simulink library "Energy_converter_Electrical_to_Mechanical"  (R2016a)
settings: Solver=ode1  StartTime=0.0  StopTime=Inf  FixedStep=0.001  RelTol=1e-3
undefined symbols (not defined in the file): API1dcac_efficiency, API2dcac_efficiency, API3dcac_efficiency, aux_power_state, AWR_InvStError, dat, DiscIntNeverNeededParam, EDCU_p_RefTqeMOT, emot_AcCmprFront_inertia, emot_AcCmprFront_nTab_3rdD, emot_AcCmprFront_pwrAC, emot_AcCmprFront_Tau, emot_AcCmprFront_trqTab_2ndD, emot_AcCmprFront_vltTab_1stD, emot_AcCmprRear_inertia, emot_AcCmprRear_nTab_3rdD, emot_AcCmprRear_pwrAC, emot_AcCmprRear_Tau, emot_AcCmprRear_trqTab_2ndD, emot_AcCmprRear_vltTab_1stD, emot_AirCmpr_inertia, emot_AirCmpr_nTab_3rdD, emot_AirCmpr_pwrAC, emot_AirCmpr_Tau, emot_AirCmpr_trqTab_2ndD, emot_AirCmpr_vltTab_1stD, emot_aircomp_power, emot_Cth_rotor, emot_Cth_stator, emot_dtrqEmotNeg, emot_dtrqEmotPtv, emot_inv_pwracTab_1st, emot_inv_pwrDC, emot_inv_pwrLoss, emot_inv_VrmsTab_2nd, emot_j, emot_mot_pwrLoss, emot_nTab_1stD, emot_pwrEtaTab_nRow, emot_pwrEtaTab_pwrTab, emot_pwrEtaTab_trqClm, emot_Rth_rotor_oil, emot_Rth_stator_oil, emot_Rth_stator_rotor, emot_tractiongroup, emot_Trotor_init, emot_trqMaxRow, emot_trqMinRow, emot_Tstator_init, emot_vltTab_3rdD, FirstDrivenAxleNoOfEmot, inv_Cth_cooling_plate, inv_Cth_diode, inv_Cth_IGBT, inv_n_IGBT_per_Switch, inv_Rth_cooling_plate_coolant, inv_Rth_PS_cooling_plate, inv_Tplate_init, inv_Tpowerstack_init, midAxleNoOfEmot ... (+6)
libraries: Electrical_converter x12, Energy_converter_Electrical_to_Mechanical x12, simulink x7
(part 5 of 8)

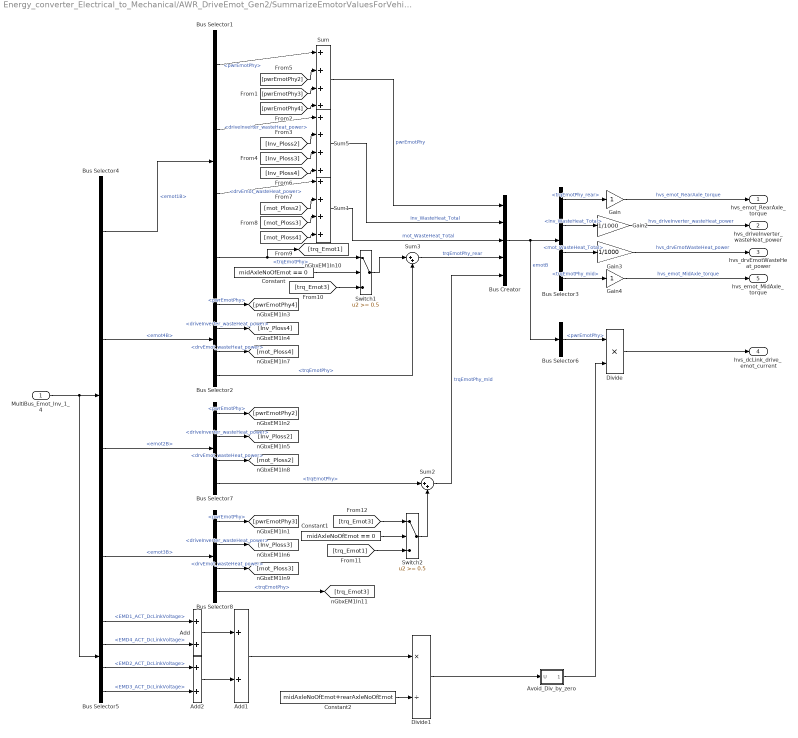
== system Energy_converter_Electrical_to_Mechanical/AWR_DriveEmot_Gen2/SummarizeEmotorValuesForVehicle ==
  MultiBus_Emot_Inv_1_4 : Inport
  Add : Sum
  Add1 : Sum
  Add2 : Sum
  Avoid_Div_by_zero : Subsystem
  Bus Creator : BusCreator  Inputs=5
  Bus Selector{1..2,7..8} (4 alike) : BusSelector  OutputSignals=pwrEmotPhy,driveInverter_wasteHeat_power,drvEmot_wasteHeat_power,trqEmotPhy
  Bus Selector3 : BusSelector  OutputSignals=trqEmotPhy_rear,Inv_WasteHeat_Total,mot_WasteHeat_Total,trqEmotPhy_mid
  Bus Selector4 : BusSelector  OutputSignals=emot1_4B.emot1B,emot1_4B.emot4B,emot2_3B.emot2B,emot2_3B.emot3B
  Bus Selector5 : BusSelector  OutputSignals=awr1_4B.awr1B.EMD1_ACT_DcLinkVoltage,awr1_4B.awr4B.EMD4_ACT_DcLinkVoltage,awr2_3B.awr2B.EMD2_ACT_DcLinkVoltage,awr2_3B.awr3B.EMD3_ACT_DcLinkVoltage
  Bus Selector6 : BusSelector  OutputSignals=pwrEmotPhy
  Constant : Constant  Value=midAxleNoOfEmot == 0
  Constant1 : Constant  Value=midAxleNoOfEmot == 0
  Constant2 : Constant  Value=midAxleNoOfEmot+rearAxleNoOfEmot
  Divide : Product  Inputs=**
  Divide1 : Product  Inputs=*/
  Gain : Gain
  Gain2 : Gain  Gain=1/1000
  Gain3 : Gain  Gain=1/1000
  Gain4 : Gain
  Sum : Sum  Inputs=|++++
  Sum1 : Sum  Inputs=|++++
  Sum2 : Sum  Inputs=|++
  Sum3 : Sum  Inputs=|++
  Sum5 : Sum  Inputs=|++++
  Switch1 : Switch  Threshold=0.5
  Switch2 : Switch  Threshold=0.5
  hvs_emot_RearAxle_torque : Outport
  hvs_driveInverter_wasteHeat_power : Outport  Port=2
  hvs_drvEmotWasteHeat_power : Outport  Port=3
  hvs_dcLink_drive_emot_current : Outport  Port=4
  hvs_emot_MidAxle_torque : Outport  Port=5
  wires:
  Add1/1 -> Divide1/1
  Constant2/1 -> Divide1/2
  [trq_Emot3] -> Switch2/1
  Switch2/1 -> Sum2/2
  [trq_Emot1] -> Switch2/3
  Constant1/1 -> Switch2/2
  [trq_Emot3] -> Switch1/3
  Switch1/1 -> Sum3/1
  Constant/1 -> Switch1/2
  Sum3/1 -> Bus Creator/4  "trqEmotPhy_rear"
  Sum1/1 -> Bus Creator/3  "mot_WasteHeat_Total"
  Sum5/1 -> Bus Creator/2  "Inv_WasteHeat_Total"
  Sum/1 -> Bus Creator/1  "pwrEmotPhy"
  Bus Selector2/4 -> Sum3/2  "<trqEmotPhy>"
  Bus Selector1/4 -> Switch1/1, [trq_Emot1]  "<trqEmotPhy>"
  Bus Selector2/3 -> [mot_Ploss4]  "<drvEmot_wasteHeat_power>"
  Bus Selector2/2 -> [Inv_Ploss4]  "<driveInverter_wasteHeat_power>"
  Bus Selector1/1 -> Sum/1  "<pwrEmotPhy>"
  Bus Selector4/2 -> Bus Selector2/1  "<emot4B>"
  Bus Selector4/1 -> Bus Selector1/1  "<emot1B>"
  MultiBus_Emot_Inv_1_4/1 -> Bus Selector5/1, Bus Selector4/1
  Bus Creator/1 -> Bus Selector6/1, Bus Selector3/1  "emotB"
  Bus Selector3/1 -> Gain/1  "<trqEmotPhy_rear>"
  Gain/1 -> hvs_emot_RearAxle_torque/1  "hvs_emot_RearAxle_torque"
  Bus Selector5/1 -> Add/1  "<EMD1_ACT_DcLinkVoltage>"
  Bus Selector5/2 -> Add/2  "<EMD4_ACT_DcLinkVoltage>"
  Divide1/1 -> Avoid_Div_by_zero/1(U)
  Bus Selector6/1 -> Divide/1  "<pwrEmotPhy>"
  Avoid_Div_by_zero/1(1/U) -> Divide/2
  Divide/1 -> hvs_dcLink_drive_emot_current/1
  Bus Selector3/2 -> Gain2/1  "<Inv_WasteHeat_Total>"
  Gain2/1 -> hvs_driveInverter_wasteHeat_power/1  "hvs_driveInverter_wasteHeat_power"
  Bus Selector3/3 -> Gain3/1  "<mot_WasteHeat_Total>"
  Gain3/1 -> hvs_drvEmotWasteHeat_power/1  "hvs_drvEmotWasteHeat_power"
  Bus Selector4/4 -> Bus Selector8/1  "<emot3B>"
  Bus Selector4/3 -> Bus Selector7/1  "<emot2B>"
  Bus Selector7/1 -> [pwrEmotPhy2]  "<pwrEmotPhy>"
  Bus Selector8/1 -> [pwrEmotPhy3]  "<pwrEmotPhy>"
  Bus Selector2/1 -> [pwrEmotPhy4]  "<pwrEmotPhy>"
  [pwrEmotPhy2] -> Sum/2
  [pwrEmotPhy3] -> Sum/3
  [pwrEmotPhy4] -> Sum/4
  [Inv_Ploss2] -> Sum5/2
  [Inv_Ploss3] -> Sum5/3
  [Inv_Ploss4] -> Sum5/4
  Bus Selector7/2 -> [Inv_Ploss2]  "<driveInverter_wasteHeat_power>"
  Bus Selector8/2 -> [Inv_Ploss3]  "<driveInverter_wasteHeat_power>"
  Bus Selector7/3 -> [mot_Ploss2]  "<drvEmot_wasteHeat_power>"
  Bus Selector8/3 -> [mot_Ploss3]  "<drvEmot_wasteHeat_power>"
  [mot_Ploss2] -> Sum1/2
  [mot_Ploss3] -> Sum1/3
  [mot_Ploss4] -> Sum1/4
  Bus Selector7/4 -> Sum2/1  "<trqEmotPhy>"
  Bus Selector8/4 -> [trq_Emot3]  "<trqEmotPhy>"
  Sum2/1 -> Bus Creator/5  "trqEmotPhy_mid"
  Bus Selector5/3 -> Add2/1  "<EMD2_ACT_DcLinkVoltage>"
  Bus Selector5/4 -> Add2/2  "<EMD3_ACT_DcLinkVoltage>"
  Gain4/1 -> hvs_emot_MidAxle_torque/1  "hvs_emot_MidAxle_torque"
  Bus Selector3/4 -> Gain4/1  "<trqEmotPhy_mid>"
  Add/1 -> Add1/1
  Add2/1 -> Add1/2
  Bus Selector1/2 -> Sum5/1  "<driveInverter_wasteHeat_power>"
  Bus Selector1/3 -> Sum1/1  "<drvEmot_wasteHeat_power>"

== system Energy_converter_Electrical_to_Mechanical/AWR_DriveEmot_Gen2/percent_to_Nm ==
  Percentage_Torque : Inport
  Reference_Torque : Inport  Port=2
  Constant : Constant  Value=100
  Divide : Product  Inputs=*/
  Product : Product  RndMeth=Zero
  Torque_Nm : Outport
  wires:
  Constant/1 -> Divide/2
  Product/1 -> Divide/1
  Reference_Torque/1 -> Product/2  "Reference_Torque"
  Divide/1 -> Torque_Nm/1  "Torque_Nm"
  Percentage_Torque/1 -> Product/1  "Percentage_Torque"

== system Energy_converter_Electrical_to_Mechanical/AWR_DriveEmot_Gen2/percent_to_Nm1 ==
  Percentage_Torque : Inport
  Reference_Torque : Inport  Port=2
  Constant : Constant  Value=100
  Divide : Product  Inputs=*/
  Product : Product  RndMeth=Zero
  Torque_Nm : Outport
  wires:
  Constant/1 -> Divide/2
  Product/1 -> Divide/1
  Reference_Torque/1 -> Product/2  "Reference_Torque"
  Divide/1 -> Torque_Nm/1  "Torque_Nm"
  Percentage_Torque/1 -> Product/1  "Percentage_Torque"

== system Energy_converter_Electrical_to_Mechanical/AWR_DriveEmot_Gen2/percent_to_Nm2 ==
  Percentage_Torque : Inport
  Reference_Torque : Inport  Port=2
  Constant : Constant  Value=100
  Divide : Product  Inputs=*/
  Product : Product  RndMeth=Zero
  Torque_Nm : Outport
  wires:
  Constant/1 -> Divide/2
  Product/1 -> Divide/1
  Reference_Torque/1 -> Product/2  "Reference_Torque"
  Divide/1 -> Torque_Nm/1  "Torque_Nm"
  Percentage_Torque/1 -> Product/1  "Percentage_Torque"

== system Energy_converter_Electrical_to_Mechanical/AWR_DriveEmot_Gen2/percent_to_Nm3 ==
  Percentage_Torque : Inport
  Reference_Torque : Inport  Port=2
  Constant : Constant  Value=100
  Divide : Product  Inputs=*/
  Product : Product  RndMeth=Zero
  Torque_Nm : Outport
  wires:
  Constant/1 -> Divide/2
  Product/1 -> Divide/1
  Reference_Torque/1 -> Product/2  "Reference_Torque"
  Divide/1 -> Torque_Nm/1  "Torque_Nm"
  Percentage_Torque/1 -> Product/1  "Percentage_Torque"

== system Energy_converter_Electrical_to_Mechanical/AWR_DriveEmot_edb_Data/AWR 1 TX ==
  IN_EMD1_ACT_DcLinkVoltage : Inport
  IN_EMD1_ACT_DigitalInput1 : Inport  Port=2
  IN_EMD1_ACT_MaximumAvailableTorque : Inport  Port=3
  IN_EMD1_ACT_DcLinkPower : Inport  Port=4
  IN_EMD1_ACT_MotorSpeed : Inport  Port=5
  IN_EMD1_ACT_Torque : Inport  Port=6
  IN_EMD1_ACT_InverterState : Inport  Port=7
  IN_EMD1_ACT_ReferenceTorqueLimited : Inport  Port=8
  IN_EMD1_ACT_MaxJunctionTemperature : Inport  Port=9
  IN_EMD1_ACT_MotorTemperature : Inport  Port=10
  IN_EMD1_ACT_InverterLosses : Inport  Port=11
  IN_EMD1_ACT_MotorLosses : Inport  Port=12
  Constant3 : Constant  Value=EDCU_p_RefTqeMOT
  Constant39 : Constant  Value=EDCU_p_RefTqeMOT
  Constant5 : Constant  Value=EDCU_p_RefTqeMOT
  Nm_to_percent : Subsystem
  Nm_to_percent1 : Subsystem
  Nm_to_percent2 : Subsystem
  hvs_EMD1_ACT_DigitalInput1 : Outport
  hvs_EMD1_ACT_InverterState : Outport  Port=2
  hvs_EMD1_ACT_MaxAvailableTorque : Outport  Port=3
  hvs_EMD1_ACT_ReferenceTorqueLim : Outport  Port=4
  hvs_EMD1_ACT_Torque : Outport  Port=5
  hvs_EMD1_ACT_DcLinkPower : Outport  Port=6
  hvs_EMD1_ACT_MotorSpeed : Outport  Port=7
  hvs_EMD1_ACT_DcLinkVoltage : Outport  Port=8
  hvs_EMD1_ACT_MaxJunctionTemp : Outport  Port=9
  hvs_EMD1_ACT_MotorTemperature : Outport  Port=10
  hvs_EMD1_ACT_InverterLosses : Outport  Port=11
  hvs_EMD1_ACT_MotorLosses : Outport  Port=12
  wires:
  Constant5/1 -> Nm_to_percent1/2(Reference_Torque)
  IN_EMD1_ACT_ReferenceTorqueLimited/1 -> Nm_to_percent1/1(Nm_Torque)  "EMD1_ACT_ReferenceTorqueLimited"
  IN_EMD1_ACT_InverterState/1 -> hvs_EMD1_ACT_InverterState/1  "hvs_EMD1_ACT_InverterState"
  IN_EMD1_ACT_DcLinkPower/1 -> hvs_EMD1_ACT_DcLinkPower/1  "hvs_EMD1_ACT_DcLinkPower"
  IN_EMD1_ACT_DcLinkVoltage/1 -> hvs_EMD1_ACT_DcLinkVoltage/1  "hvs_EMD1_ACT_DcLinkVoltage"
  Nm_to_percent/1(Torque_Percentage) -> hvs_EMD1_ACT_MaxAvailableTorque/1  "hvs_EMD1_ACT_MaxAvailableTorque"
  Nm_to_percent1/1(Torque_Percentage) -> hvs_EMD1_ACT_ReferenceTorqueLim/1  "hvs_EMD1_ACT_ReferenceTorqueLim"
  IN_EMD1_ACT_MotorSpeed/1 -> hvs_EMD1_ACT_MotorSpeed/1  "hvs_EMD1_ACT_MotorSpeed"
  IN_EMD1_ACT_Torque/1 -> Nm_to_percent2/1(Nm_Torque)
  IN_EMD1_ACT_MaxJunctionTemperature/1 -> hvs_EMD1_ACT_MaxJunctionTemp/1  "hvs_EMD1_ACT_MaxJunctionTemp"
  IN_EMD1_ACT_MotorTemperature/1 -> hvs_EMD1_ACT_MotorTemperature/1  "hvs_EMD1_ACT_MotorTemperature"
  IN_EMD1_ACT_DigitalInput1/1 -> hvs_EMD1_ACT_DigitalInput1/1  "hvs_EMD1_ACT_DigitalInput1"
  IN_EMD1_ACT_MaximumAvailableTorque/1 -> Nm_to_percent/1(Nm_Torque)  "EMD1_ACT_MaximumAvailableTorque"
  Constant3/1 -> Nm_to_percent/2(Reference_Torque)
  Nm_to_percent2/1(Torque_Percentage) -> hvs_EMD1_ACT_Torque/1  "hvs_EMD1_ACT_Torque"
  Constant39/1 -> Nm_to_percent2/2(Reference_Torque)
  IN_EMD1_ACT_InverterLosses/1 -> hvs_EMD1_ACT_InverterLosses/1  "hvs_EMD1_ACT_InverterLosses"
  IN_EMD1_ACT_MotorLosses/1 -> hvs_EMD1_ACT_MotorLosses/1  "hvs_EMD1_ACT_MotorLosses"

== system Energy_converter_Electrical_to_Mechanical/AWR_DriveEmot_edb_Data/AWR 2 TX ==
  IN_EMD2_ACT_DcLinkVoltage : Inport
  IN_EMD2_ACT_DigitalInput1 : Inport  Port=2
  IN_EMD2_ACT_MaximumAvailableTorque : Inport  Port=3
  IN_EMD2_ACT_DcLinkPower : Inport  Port=4
  IN_EMD2_ACT_MotorSpeed : Inport  Port=5
  IN_EMD2_ACT_Torque : Inport  Port=6
  IN_EMD2_ACT_InverterState : Inport  Port=7
  IN_EMD2_ACT_ReferenceTorqueLimited : Inport  Port=8
  IN_EMD2_ACT_MaxJunctionTemperature : Inport  Port=9
  IN_EMD2_ACT_MotorTemperature : Inport  Port=10
  IN_EMD2_ACT_InverterLosses : Inport  Port=11
  IN_EMD2_ACT_MotorLosses : Inport  Port=12
  Constant3 : Constant  Value=EDCU_p_RefTqeMOT
  Constant39 : Constant  Value=EDCU_p_RefTqeMOT
  Constant5 : Constant  Value=EDCU_p_RefTqeMOT
  Nm_to_percent : Subsystem
  Nm_to_percent1 : Subsystem
  Nm_to_percent2 : Subsystem
  hvs_EMD2_ACT_DigitalInput1 : Outport
  hvs_EMD2_ACT_InverterState : Outport  Port=2
  hvs_EMD2_ACT_MaxAvailableTorque : Outport  Port=3
  hvs_EMD2_ACT_ReferenceTorqueLim : Outport  Port=4
  hvs_EMD2_ACT_Torque : Outport  Port=5
  hvs_EMD2_ACT_DcLinkPower : Outport  Port=6
  hvs_EMD2_ACT_MotorSpeed : Outport  Port=7
  hvs_EMD2_ACT_DcLinkVoltage : Outport  Port=8
  hvs_EMD2_ACT_MaxJunctionTemp : Outport  Port=9
  hvs_EMD2_ACT_MotorTemperature : Outport  Port=10
  hvs_EMD2_ACT_InverterLosses : Outport  Port=11
  hvs_EMD2_ACT_MotorLosses : Outport  Port=12
  wires:
  Constant5/1 -> Nm_to_percent1/2(Reference_Torque)
  IN_EMD2_ACT_ReferenceTorqueLimited/1 -> Nm_to_percent1/1(Nm_Torque)  "EMD1_ACT_ReferenceTorqueLimited"
  IN_EMD2_ACT_InverterState/1 -> hvs_EMD2_ACT_InverterState/1  "hvs_EMD2_ACT_InverterState"
  IN_EMD2_ACT_DcLinkPower/1 -> hvs_EMD2_ACT_DcLinkPower/1  "hvs_EMD2_ACT_DcLinkPower"
  IN_EMD2_ACT_DcLinkVoltage/1 -> hvs_EMD2_ACT_DcLinkVoltage/1  "hvs_EMD2_ACT_DcLinkVoltage"
  Nm_to_percent/1(Torque_Percentage) -> hvs_EMD2_ACT_MaxAvailableTorque/1  "hvs_EMD2_ACT_MaxAvailableTorque"
  Nm_to_percent1/1(Torque_Percentage) -> hvs_EMD2_ACT_ReferenceTorqueLim/1  "hvs_EMD2_ACT_ReferenceTorqueLim"
  IN_EMD2_ACT_MotorSpeed/1 -> hvs_EMD2_ACT_MotorSpeed/1  "hvs_EMD2_ACT_MotorSpeed"
  IN_EMD2_ACT_Torque/1 -> Nm_to_percent2/1(Nm_Torque)
  IN_EMD2_ACT_MaxJunctionTemperature/1 -> hvs_EMD2_ACT_MaxJunctionTemp/1  "hvs_EMD2_ACT_MaxJunctionTemp"
  IN_EMD2_ACT_MotorTemperature/1 -> hvs_EMD2_ACT_MotorTemperature/1  "hvs_EMD2_ACT_MotorTemperature"
  IN_EMD2_ACT_DigitalInput1/1 -> hvs_EMD2_ACT_DigitalInput1/1  "hvs_EMD2_ACT_DigitalInput1"
  IN_EMD2_ACT_MaximumAvailableTorque/1 -> Nm_to_percent/1(Nm_Torque)  "EMD1_ACT_MaximumAvailableTorque"
  Constant3/1 -> Nm_to_percent/2(Reference_Torque)
  Nm_to_percent2/1(Torque_Percentage) -> hvs_EMD2_ACT_Torque/1  "hvs_EMD2_ACT_Torque"
  Constant39/1 -> Nm_to_percent2/2(Reference_Torque)
  IN_EMD2_ACT_InverterLosses/1 -> hvs_EMD2_ACT_InverterLosses/1  "hvs_EMD2_ACT_InverterLosses"
  IN_EMD2_ACT_MotorLosses/1 -> hvs_EMD2_ACT_MotorLosses/1  "hvs_EMD2_ACT_MotorLosses"

== system Energy_converter_Electrical_to_Mechanical/AWR_DriveEmot_edb_Data/AWR 3 TX ==
  IN_EMD3_ACT_DcLinkVoltage : Inport
  IN_EMD3_ACT_DigitalInput1 : Inport  Port=2
  IN_EMD3_ACT_MaximumAvailableTorque : Inport  Port=3
  IN_EMD3_ACT_DcLinkPower : Inport  Port=4
  IN_EMD3_ACT_MotorSpeed : Inport  Port=5
  IN_EMD3_ACT_Torque : Inport  Port=6
  IN_EMD3_ACT_InverterState : Inport  Port=7
  IN_EMD3_ACT_ReferenceTorqueLimited : Inport  Port=8
  IN_EMD3_ACT_MaxJunctionTemperature : Inport  Port=9
  IN_EMD3_ACT_MotorTemperature : Inport  Port=10
  IN_EMD3_ACT_InverterLosses : Inport  Port=11
  IN_EMD3_ACT_MotorLosses : Inport  Port=12
  Constant3 : Constant  Value=EDCU_p_RefTqeMOT
  Constant39 : Constant  Value=EDCU_p_RefTqeMOT
  Constant5 : Constant  Value=EDCU_p_RefTqeMOT
  Nm_to_percent : Subsystem
  Nm_to_percent1 : Subsystem
  Nm_to_percent2 : Subsystem
  hvs_EMD3_ACT_DigitalInput1 : Outport
  hvs_EMD3_ACT_InverterState : Outport  Port=2
  hvs_EMD3_ACT_MaxAvailableTorque : Outport  Port=3
  hvs_EMD3_ACT_ReferenceTorqueLim : Outport  Port=4
  hvs_EMD3_ACT_Torque : Outport  Port=5
  hvs_EMD3_ACT_DcLinkPower : Outport  Port=6
  hvs_EMD3_ACT_MotorSpeed : Outport  Port=7
  hvs_EMD3_ACT_DcLinkVoltage : Outport  Port=8
  hvs_EMD3_ACT_MaxJunctionTemp : Outport  Port=9
  hvs_EMD3_ACT_MotorTemperature : Outport  Port=10
  hvs_EMD3_ACT_InverterLosses : Outport  Port=11
  hvs_EMD3_ACT_MotorLosses : Outport  Port=12
  wires:
  Constant39/1 -> Nm_to_percent2/2(Reference_Torque)
  Nm_to_percent2/1(Torque_Percentage) -> hvs_EMD3_ACT_Torque/1  "hvs_EMD3_ACT_Torque"
  Constant3/1 -> Nm_to_percent/2(Reference_Torque)
  IN_EMD3_ACT_MaximumAvailableTorque/1 -> Nm_to_percent/1(Nm_Torque)  "EMD1_ACT_MaximumAvailableTorque"
  IN_EMD3_ACT_DigitalInput1/1 -> hvs_EMD3_ACT_DigitalInput1/1  "hvs_EMD3_ACT_DigitalInput1"
  IN_EMD3_ACT_MotorTemperature/1 -> hvs_EMD3_ACT_MotorTemperature/1  "hvs_EMD3_ACT_MotorTemperature"
  IN_EMD3_ACT_MaxJunctionTemperature/1 -> hvs_EMD3_ACT_MaxJunctionTemp/1  "hvs_EMD3_ACT_MaxJunctionTemp"
  IN_EMD3_ACT_Torque/1 -> Nm_to_percent2/1(Nm_Torque)
  IN_EMD3_ACT_MotorSpeed/1 -> hvs_EMD3_ACT_MotorSpeed/1  "hvs_EMD3_ACT_MotorSpeed"
  Nm_to_percent1/1(Torque_Percentage) -> hvs_EMD3_ACT_ReferenceTorqueLim/1  "hvs_EMD3_ACT_ReferenceTorqueLim"
  Nm_to_percent/1(Torque_Percentage) -> hvs_EMD3_ACT_MaxAvailableTorque/1  "hvs_EMD3_ACT_MaxAvailableTorque"
  IN_EMD3_ACT_DcLinkVoltage/1 -> hvs_EMD3_ACT_DcLinkVoltage/1  "hvs_EMD3_ACT_DcLinkVoltage"
  IN_EMD3_ACT_DcLinkPower/1 -> hvs_EMD3_ACT_DcLinkPower/1  "hvs_EMD3_ACT_DcLinkPower"
  IN_EMD3_ACT_InverterState/1 -> hvs_EMD3_ACT_InverterState/1  "hvs_EMD3_ACT_InverterState"
  IN_EMD3_ACT_ReferenceTorqueLimited/1 -> Nm_to_percent1/1(Nm_Torque)  "EMD1_ACT_ReferenceTorqueLimited"
  Constant5/1 -> Nm_to_percent1/2(Reference_Torque)
  IN_EMD3_ACT_InverterLosses/1 -> hvs_EMD3_ACT_InverterLosses/1  "hvs_EMD3_ACT_InverterLosses"
  IN_EMD3_ACT_MotorLosses/1 -> hvs_EMD3_ACT_MotorLosses/1  "hvs_EMD3_ACT_MotorLosses"

== system Energy_converter_Electrical_to_Mechanical/AWR_DriveEmot_edb_Data/AWR 4 TX ==
  IN_EMD4_ACT_DcLinkVoltage : Inport
  IN_EMD4_ACT_DigitalInput1 : Inport  Port=2
  IN_EMD4_ACT_MaximumAvailableTorque : Inport  Port=3
  IN_EMD4_ACT_DcLinkPower : Inport  Port=4
  IN_EMD4_ACT_MotorSpeed : Inport  Port=5
  IN_EMD4_ACT_Torque : Inport  Port=6
  IN_EMD4_ACT_InverterState : Inport  Port=7
  IN_EMD4_ACT_ReferenceTorqueLimited : Inport  Port=8
  IN_EMD4_ACT_MaxJunctionTemperature : Inport  Port=9
  IN_EMD4_ACT_MotorTemperature : Inport  Port=10
  IN_EMD4_ACT_InverterLosses : Inport  Port=11
  IN_EMD4_ACT_MotorLosses : Inport  Port=12
  Constant3 : Constant  Value=EDCU_p_RefTqeMOT
  Constant39 : Constant  Value=EDCU_p_RefTqeMOT
  Constant5 : Constant  Value=EDCU_p_RefTqeMOT
  Nm_to_percent : Subsystem
  Nm_to_percent1 : Subsystem
  Nm_to_percent2 : Subsystem
  hvs_EMD4_ACT_DigitalInput1 : Outport
  hvs_EMD4_ACT_InverterState : Outport  Port=2
  hvs_EMD4_ACT_MaxAvailableTorque : Outport  Port=3
  hvs_EMD4_ACT_ReferenceTorqueLim : Outport  Port=4
  hvs_EMD4_ACT_Torque : Outport  Port=5
  hvs_EMD4_ACT_DcLinkPower : Outport  Port=6
  hvs_EMD4_ACT_MotorSpeed : Outport  Port=7
  hvs_EMD4_ACT_DcLinkVoltage : Outport  Port=8
  hvs_EMD4_ACT_MaxJunctionTemperature : Outport  Port=9
  hvs_EMD4_ACT_MotorTemperature : Outport  Port=10
  hvs_EMD4_ACT_InverterLosses : Outport  Port=11
  hvs_EMD4_ACT_MotorLosses : Outport  Port=12
  wires:
  Constant5/1 -> Nm_to_percent1/2(Reference_Torque)
  IN_EMD4_ACT_ReferenceTorqueLimited/1 -> Nm_to_percent1/1(Nm_Torque)  "EMD4_ACT_ReferenceTorqueLimited"
  IN_EMD4_ACT_InverterState/1 -> hvs_EMD4_ACT_InverterState/1  "hvs_EMD4_ACT_InverterState"
  IN_EMD4_ACT_DcLinkPower/1 -> hvs_EMD4_ACT_DcLinkPower/1  "hvs_EMD4_ACT_DcLinkPower"
  IN_EMD4_ACT_DcLinkVoltage/1 -> hvs_EMD4_ACT_DcLinkVoltage/1  "hvs_EMD4_ACT_DcLinkVoltage"
  Nm_to_percent/1(Torque_Percentage) -> hvs_EMD4_ACT_MaxAvailableTorque/1  "hvs_EMD4_ACT_MaxAvailableTorque"
  IN_EMD4_ACT_MotorSpeed/1 -> hvs_EMD4_ACT_MotorSpeed/1  "hvs_EMD4_ACT_MotorSpeed"
  IN_EMD4_ACT_Torque/1 -> Nm_to_percent2/1(Nm_Torque)
  IN_EMD4_ACT_MaxJunctionTemperature/1 -> hvs_EMD4_ACT_MaxJunctionTemperature/1  "hvs_EMD4_ACT_MaxJunctionTemperature"
  IN_EMD4_ACT_MotorTemperature/1 -> hvs_EMD4_ACT_MotorTemperature/1  "hvs_EMD4_ACT_MotorTemperature"
  Nm_to_percent1/1(Torque_Percentage) -> hvs_EMD4_ACT_ReferenceTorqueLim/1  "hvs_EMD4_ACT_ReferenceTorqueLim"
  IN_EMD4_ACT_DigitalInput1/1 -> hvs_EMD4_ACT_DigitalInput1/1  "hvs_EMD4_ACT_DigitalInput1"
  IN_EMD4_ACT_MaximumAvailableTorque/1 -> Nm_to_percent/1(Nm_Torque)  "EMD2_ACT_MaximumAvailableTorque"
  Constant3/1 -> Nm_to_percent/2(Reference_Torque)
  Constant39/1 -> Nm_to_percent2/2(Reference_Torque)
  Nm_to_percent2/1(Torque_Percentage) -> hvs_EMD4_ACT_Torque/1  "hvs_EMD4_ACT_Torque"
  IN_EMD4_ACT_InverterLosses/1 -> hvs_EMD4_ACT_InverterLosses/1  "hvs_EMD4_ACT_InverterLosses"
  IN_EMD4_ACT_MotorLosses/1 -> hvs_EMD4_ACT_MotorLosses/1  "hvs_EMD4_ACT_MotorLosses"

== system Energy_converter_Electrical_to_Mechanical/AWR_DriveEmot_edb_Data/AWR1_4 ==
  EMD1_CMD_Commamd : Inport
  EMD1_CMD_MotorControlMode : Inport  Port=2
  EMD1_CMD_SpeedRefLim : Inport  Port=3
  EMD1_CMD_TorqueRefLim : Inport  Port=4
  HVFreigabeHW_SiRelay_D : Inport  Port=5
  vltZkBmsPhy : Inport  Port=6
  trqEmot1Phy : Inport  Port=7
  trqEmot4Phy : Inport  Port=8
  pwEmot1Phy : Inport  Port=9
  pwEmot4Phy : Inport  Port=10
  trqEmot1Max : Inport  Port=11
  trqEmot4Max : Inport  Port=12
  nGbxEMIn : Inport  Port=13
  EMD4_CMD_Commamd : Inport  Port=14
  EMD4_CMD_MotorControlMode : Inport  Port=15
  EMD4_CMD_SpeedRefLim : Inport  Port=16
  EMD4_CMD_TorqueRefLim : Inport  Port=17
  HVFreigabeHW4_SiRelay_D : Inport  Port=18
  EDCU_Dig_SafetyCutOffDG1 : Inport  Port=19
  Bus Creator3 : BusCreator  Inputs=11
  Bus Creator4 : BusCreator  Inputs=2
  Bus Creator5 : BusCreator  Inputs=11
  Gain : Gain
  Gain1 : Gain
  Switch1 : Switch  Threshold=0.5
  Switch2 : Switch  Threshold=0.5
  ZeroWhenNotReady1 : Subsystem  TreatAsAtomicUnit=on
  ZeroWhenNotReady2 : Subsystem  TreatAsAtomicUnit=on
  awr : Electrical_converter/awr  SystemSampleTime=-1
  awr1 : Electrical_converter/awr  SystemSampleTime=-1
  awr1_4B : Outport
  wires:
  nGbxEMIn/1 -> [nGbxEMIn], awr/10
  vltZkBmsPhy/1 -> [vltZkBmsPhy], awr/6
  EMD1_CMD_MotorControlMode/1 -> awr/2
  EMD4_CMD_MotorControlMode/1 -> awr1/2
  [nGbxEMIn] -> awr1/10
  Gain1/1 -> Bus Creator3/1  "EMD4_ACT_DcLinkVoltage"
  Gain/1 -> Bus Creator5/1  "EMD1_ACT_DcLinkVoltage"
  EMD1_CMD_SpeedRefLim/1 -> awr/3
  EMD1_CMD_TorqueRefLim/1 -> awr/4
  HVFreigabeHW_SiRelay_D/1 -> awr/5
  HVFreigabeHW4_SiRelay_D/1 -> awr1/5
  EMD4_CMD_SpeedRefLim/1 -> awr1/3
  EMD4_CMD_Commamd/1 -> awr1/1
  EMD4_CMD_TorqueRefLim/1 -> awr1/4
  Bus Creator4/1 -> awr1_4B/1  "awr1_4B"
  trqEmot4Phy/1 -> awr1/7
  pwEmot4Phy/1 -> awr1/8
  trqEmot4Max/1 -> awr1/9
  trqEmot1Phy/1 -> awr/7
  pwEmot1Phy/1 -> awr/8
  trqEmot1Max/1 -> awr/9
  Bus Creator3/1 -> Switch1/1  "awr4B"
  ZeroWhenNotReady2/1(Out1) -> Switch1/3
  Switch1/1 -> Bus Creator4/2  "awr4B"
  awr1/2 -> Bus Creator3/2
  awr1/3 -> Bus Creator3/3
  awr1/10 -> Bus Creator3/10
  awr1/11 -> Bus Creator3/11
  awr1/5 -> Bus Creator3/5
  awr1/9 -> Bus Creator3/9
  awr1/8 -> Bus Creator3/8
  awr1/7 -> Bus Creator3/7
  awr1/6 -> Bus Creator3/6
  awr1/1 -> Gain1/1
  awr1/4 -> Bus Creator3/4
  ZeroWhenNotReady1/1(Out1) -> Switch2/3
  Switch2/1 -> Bus Creator4/1  "awr1B"
  awr1/12 -> Switch1/2
  awr/9 -> Bus Creator5/9
  awr/7 -> Bus Creator5/7
  awr/6 -> Bus Creator5/6
  awr/10 -> Bus Creator5/10
  awr/11 -> Bus Creator5/11
  awr/8 -> Bus Creator5/8
  awr/5 -> Bus Creator5/5
  awr/4 -> Bus Creator5/4
  awr/1 -> Gain/1
  awr/3 -> Bus Creator5/3
  awr/2 -> Bus Creator5/2
  awr/12 -> Switch2/2
  Bus Creator5/1 -> Switch2/1
  EMD1_CMD_Commamd/1 -> awr/1
  [vltZkBmsPhy] -> awr1/6
  EDCU_Dig_SafetyCutOffDG1/1 -> [EDCU_Dig_SafetyCutOffDG1], awr/11
  [EDCU_Dig_SafetyCutOffDG1] -> awr1/11

== system Energy_converter_Electrical_to_Mechanical/AWR_DriveEmot_edb_Data/AWR2_3 ==
  EMD2_CMD_Commamd : Inport
  EMD2_CMD_MotorControlMode : Inport  Port=2
  EMD2_CMD_SpeedRefLim : Inport  Port=3
  EMD2_CMD_TorqueRefLim : Inport  Port=4
  HVFreigabeHW2_SiRelay_D : Inport  Port=5
  vltZkBmsPhy : Inport  Port=6
  trqEmot2Phy : Inport  Port=7
  trqEmot3Phy : Inport  Port=8
  pwEmot2Phy : Inport  Port=9
  pwEmot3Phy : Inport  Port=10
  trqEmot2Max : Inport  Port=11
  trqEmot3Max : Inport  Port=12
  nGbxEMIn : Inport  Port=13
  EMD3_CMD_Commamd : Inport  Port=14
  EMD3_CMD_MotorControlMode : Inport  Port=15
  EMD3_CMD_SpeedRefLim : Inport  Port=16
  EMD3_CMD_TorqueRefLim : Inport  Port=17
  HVFreigabeHW3_SiRelay_D : Inport  Port=18
  EDCU_Dig_SafetyCutOffDG1 : Inport  Port=19
  Enable : EnablePort  StatesWhenEnabling=reset
  Bus Creator3 : BusCreator  Inputs=11
  Bus Creator4 : BusCreator  Inputs=2
  Bus Creator5 : BusCreator  Inputs=11
  Gain : Gain
  Gain1 : Gain
  Switch1 : Switch  Threshold=0.5
  Switch2 : Switch  Threshold=0.5
  ZeroWhenNotReady1 : Subsystem  TreatAsAtomicUnit=on
  ZeroWhenNotReady2 : Subsystem  TreatAsAtomicUnit=on
  awr : Electrical_converter/awr  SystemSampleTime=-1
  awr1 : Electrical_converter/awr  SystemSampleTime=-1
  awr2_3B : Outport
  wires:
  [vltZkBmsPhy] -> awr1/6
  EMD2_CMD_Commamd/1 -> awr/1
  Bus Creator5/1 -> Switch2/1
  awr/12 -> Switch2/2
  awr/2 -> Bus Creator5/2
  awr/3 -> Bus Creator5/3
  awr/1 -> Gain/1
  awr/4 -> Bus Creator5/4
  awr/5 -> Bus Creator5/5
  awr/8 -> Bus Creator5/8
  awr/11 -> Bus Creator5/11
  awr/10 -> Bus Creator5/10
  awr/6 -> Bus Creator5/6
  awr/7 -> Bus Creator5/7
  awr/9 -> Bus Creator5/9
  awr1/12 -> Switch1/2
  Switch2/1 -> Bus Creator4/1  "awr2B"
  ZeroWhenNotReady1/1(Out1) -> Switch2/3
  awr1/4 -> Bus Creator3/4
  awr1/1 -> Gain1/1
  awr1/6 -> Bus Creator3/6
  awr1/7 -> Bus Creator3/7
  awr1/8 -> Bus Creator3/8
  awr1/9 -> Bus Creator3/9
  awr1/5 -> Bus Creator3/5
  awr1/11 -> Bus Creator3/11
  awr1/10 -> Bus Creator3/10
  awr1/3 -> Bus Creator3/3
  awr1/2 -> Bus Creator3/2
  Switch1/1 -> Bus Creator4/2  "awr3B"
  ZeroWhenNotReady2/1(Out1) -> Switch1/3
  Bus Creator3/1 -> Switch1/1  "awr4B"
  trqEmot2Max/1 -> awr/9
  pwEmot2Phy/1 -> awr/8
  trqEmot2Phy/1 -> awr/7
  trqEmot3Max/1 -> awr1/9
  pwEmot3Phy/1 -> awr1/8
  trqEmot3Phy/1 -> awr1/7
  Bus Creator4/1 -> awr2_3B/1  "awr2_3B"
  EMD3_CMD_TorqueRefLim/1 -> awr1/4
  EMD3_CMD_Commamd/1 -> awr1/1
  EMD3_CMD_SpeedRefLim/1 -> awr1/3
  HVFreigabeHW3_SiRelay_D/1 -> awr1/5
  HVFreigabeHW2_SiRelay_D/1 -> awr/5
  EMD2_CMD_TorqueRefLim/1 -> awr/4
  EMD2_CMD_SpeedRefLim/1 -> awr/3
  Gain/1 -> Bus Creator5/1  "EMD2_ACT_DcLinkVoltage"
  Gain1/1 -> Bus Creator3/1  "EMD3_ACT_DcLinkVoltage"
  [nGbxEMIn] -> awr1/10
  EMD3_CMD_MotorControlMode/1 -> awr1/2
  EMD2_CMD_MotorControlMode/1 -> awr/2
  vltZkBmsPhy/1 -> awr/6, [vltZkBmsPhy]
  nGbxEMIn/1 -> awr/10, [nGbxEMIn]
  EDCU_Dig_SafetyCutOffDG1/1 -> [EDCU_Dig_SafetyCutOffDG1], awr/11
  [EDCU_Dig_SafetyCutOffDG1] -> awr1/11

== system Energy_converter_Electrical_to_Mechanical/AWR_DriveEmot_edb_Data/EMD1_CMD_Command ==
  EMD1_CMD_ClearErrors : Inport
  EMD1_CMD_MotorControlMode : Inport  Port=2
  Compare To Constant : Subsystem  mask(Compare To Constant){relop===, const=1, OutDataTypeStr=boolean, ZeroCross=on}
      mask prompts: relop "Simulink:masks:Operator_MP"; const "Simulink:masks:ConstantValue_MP"; OutDataTypeStr "Simulink:masks:OutputDataType_MP"; ZeroCross "Simulink:masks:EnableZerocrossingDetection_MP"
      mask help: Simulink:masks:CompareToConstant_MD
      mask init: same as Energy_converter_Electrical_to_Mechanical/AWR_DriveEmot/EMD1_CMD_Command/Compare To Constant
      mask TypeOptions relop: == | ~= | < | <= | >= | >
      mask TypeOptions OutDataTypeStr: Simulink:masks:uint8 | Simulink:masks:boolean
      mask Callback ZeroCross: sl('zeroCrossEnable', gcbh);
      mask Display: disp(str)
  Compare To Constant1 : Subsystem  mask(Compare To Constant){relop===, const=1, OutDataTypeStr=boolean, ZeroCross=on}
      mask prompts: relop "Simulink:masks:Operator_MP"; const "Simulink:masks:ConstantValue_MP"; OutDataTypeStr "Simulink:masks:OutputDataType_MP"; ZeroCross "Simulink:masks:EnableZerocrossingDetection_MP"
      mask help: Simulink:masks:CompareToConstant_MD
      mask init: same as Energy_converter_Electrical_to_Mechanical/AWR_DriveEmot/EMD1_CMD_Command/Compare To Constant
      mask TypeOptions relop: == | ~= | < | <= | >= | >
      mask TypeOptions OutDataTypeStr: Simulink:masks:uint8 | Simulink:masks:boolean
      mask Callback ZeroCross: sl('zeroCrossEnable', gcbh);
      mask Display: disp(str)
  Constant : Constant  Value=4
  Constant3 : Constant
  Constant4 : Constant  Value=0
  Switch : Switch  Threshold=0.5
  Switch1 : Switch  Threshold=0.5
  Out_EMD1_CMD_Command : Outport
  wires:
  Compare To Constant/1(y) -> Switch1/2
  Switch/1 -> Out_EMD1_CMD_Command/1
  Constant4/1 -> Switch1/3
  Constant3/1 -> Switch1/1
  Constant/1 -> Switch/1
  Switch1/1 -> Switch/3
  Compare To Constant1/1(y) -> Switch/2
  EMD1_CMD_ClearErrors/1 -> Compare To Constant1/1(u)
  EMD1_CMD_MotorControlMode/1 -> Compare To Constant/1(u)

== system Energy_converter_Electrical_to_Mechanical/AWR_DriveEmot_edb_Data/EMD1_CMD_Command1 ==
  EMD1_CMD_ClearErrors : Inport
  EMD1_CMD_MotorControlMode : Inport  Port=2
  Compare To Constant : Subsystem  mask(Compare To Constant){relop===, const=1, OutDataTypeStr=boolean, ZeroCross=on}
      mask prompts: relop "Simulink:masks:Operator_MP"; const "Simulink:masks:ConstantValue_MP"; OutDataTypeStr "Simulink:masks:OutputDataType_MP"; ZeroCross "Simulink:masks:EnableZerocrossingDetection_MP"
      mask help: Simulink:masks:CompareToConstant_MD
      mask init: same as Energy_converter_Electrical_to_Mechanical/AWR_DriveEmot/EMD1_CMD_Command/Compare To Constant
      mask TypeOptions relop: == | ~= | < | <= | >= | >
      mask TypeOptions OutDataTypeStr: Simulink:masks:uint8 | Simulink:masks:boolean
      mask Callback ZeroCross: sl('zeroCrossEnable', gcbh);
      mask Display: disp(str)
  Compare To Constant1 : Subsystem  mask(Compare To Constant){relop===, const=1, OutDataTypeStr=boolean, ZeroCross=on}
      mask prompts: relop "Simulink:masks:Operator_MP"; const "Simulink:masks:ConstantValue_MP"; OutDataTypeStr "Simulink:masks:OutputDataType_MP"; ZeroCross "Simulink:masks:EnableZerocrossingDetection_MP"
      mask help: Simulink:masks:CompareToConstant_MD
      mask init: same as Energy_converter_Electrical_to_Mechanical/AWR_DriveEmot/EMD1_CMD_Command/Compare To Constant
      mask TypeOptions relop: == | ~= | < | <= | >= | >
      mask TypeOptions OutDataTypeStr: Simulink:masks:uint8 | Simulink:masks:boolean
      mask Callback ZeroCross: sl('zeroCrossEnable', gcbh);
      mask Display: disp(str)
  Constant : Constant  Value=4
  Constant3 : Constant
  Constant4 : Constant  Value=0
  Switch : Switch  Threshold=0.5
  Switch1 : Switch  Threshold=0.5
  Out_EMD1_CMD_Command : Outport
  wires:
  Compare To Constant/1(y) -> Switch1/2
  Switch/1 -> Out_EMD1_CMD_Command/1
  Constant4/1 -> Switch1/3
  Constant3/1 -> Switch1/1
  Constant/1 -> Switch/1
  Switch1/1 -> Switch/3
  Compare To Constant1/1(y) -> Switch/2
  EMD1_CMD_ClearErrors/1 -> Compare To Constant1/1(u)
  EMD1_CMD_MotorControlMode/1 -> Compare To Constant/1(u)

== system Energy_converter_Electrical_to_Mechanical/AWR_DriveEmot_edb_Data/EMD1_CMD_Command2 ==
  EMD1_CMD_ClearErrors : Inport
  EMD1_CMD_MotorControlMode : Inport  Port=2
  Compare To Constant : Subsystem  mask(Compare To Constant){relop===, const=1, OutDataTypeStr=boolean, ZeroCross=on}
      mask prompts: relop "Simulink:masks:Operator_MP"; const "Simulink:masks:ConstantValue_MP"; OutDataTypeStr "Simulink:masks:OutputDataType_MP"; ZeroCross "Simulink:masks:EnableZerocrossingDetection_MP"
      mask help: Simulink:masks:CompareToConstant_MD
      mask init: same as Energy_converter_Electrical_to_Mechanical/AWR_DriveEmot/EMD1_CMD_Command/Compare To Constant
      mask TypeOptions relop: == | ~= | < | <= | >= | >
      mask TypeOptions OutDataTypeStr: Simulink:masks:uint8 | Simulink:masks:boolean
      mask Callback ZeroCross: sl('zeroCrossEnable', gcbh);
      mask Display: disp(str)
  Compare To Constant1 : Subsystem  mask(Compare To Constant){relop===, const=1, OutDataTypeStr=boolean, ZeroCross=on}
      mask prompts: relop "Simulink:masks:Operator_MP"; const "Simulink:masks:ConstantValue_MP"; OutDataTypeStr "Simulink:masks:OutputDataType_MP"; ZeroCross "Simulink:masks:EnableZerocrossingDetection_MP"
      mask help: Simulink:masks:CompareToConstant_MD
      mask init: same as Energy_converter_Electrical_to_Mechanical/AWR_DriveEmot/EMD1_CMD_Command/Compare To Constant
      mask TypeOptions relop: == | ~= | < | <= | >= | >
      mask TypeOptions OutDataTypeStr: Simulink:masks:uint8 | Simulink:masks:boolean
      mask Callback ZeroCross: sl('zeroCrossEnable', gcbh);
      mask Display: disp(str)
  Constant : Constant  Value=4
  Constant3 : Constant
  Constant4 : Constant  Value=0
  Switch : Switch  Threshold=0.5
  Switch1 : Switch  Threshold=0.5
  Out_EMD1_CMD_Command : Outport
  wires:
  Compare To Constant/1(y) -> Switch1/2
  Switch/1 -> Out_EMD1_CMD_Command/1
  Constant4/1 -> Switch1/3
  Constant3/1 -> Switch1/1
  Constant/1 -> Switch/1
  Switch1/1 -> Switch/3
  Compare To Constant1/1(y) -> Switch/2
  EMD1_CMD_ClearErrors/1 -> Compare To Constant1/1(u)
  EMD1_CMD_MotorControlMode/1 -> Compare To Constant/1(u)

== system Energy_converter_Electrical_to_Mechanical/AWR_DriveEmot_edb_Data/EMD1_CMD_Command3 ==
  EMD1_CMD_ClearErrors : Inport
  EMD1_CMD_MotorControlMode : Inport  Port=2
  Compare To Constant : Subsystem  mask(Compare To Constant){relop===, const=1, OutDataTypeStr=boolean, ZeroCross=on}
      mask prompts: relop "Simulink:masks:Operator_MP"; const "Simulink:masks:ConstantValue_MP"; OutDataTypeStr "Simulink:masks:OutputDataType_MP"; ZeroCross "Simulink:masks:EnableZerocrossingDetection_MP"
      mask help: Simulink:masks:CompareToConstant_MD
      mask init: same as Energy_converter_Electrical_to_Mechanical/AWR_DriveEmot/EMD1_CMD_Command/Compare To Constant
      mask TypeOptions relop: == | ~= | < | <= | >= | >
      mask TypeOptions OutDataTypeStr: Simulink:masks:uint8 | Simulink:masks:boolean
      mask Callback ZeroCross: sl('zeroCrossEnable', gcbh);
      mask Display: disp(str)
  Compare To Constant1 : Subsystem  mask(Compare To Constant){relop===, const=1, OutDataTypeStr=boolean, ZeroCross=on}
      mask prompts: relop "Simulink:masks:Operator_MP"; const "Simulink:masks:ConstantValue_MP"; OutDataTypeStr "Simulink:masks:OutputDataType_MP"; ZeroCross "Simulink:masks:EnableZerocrossingDetection_MP"
      mask help: Simulink:masks:CompareToConstant_MD
      mask init: same as Energy_converter_Electrical_to_Mechanical/AWR_DriveEmot/EMD1_CMD_Command/Compare To Constant
      mask TypeOptions relop: == | ~= | < | <= | >= | >
      mask TypeOptions OutDataTypeStr: Simulink:masks:uint8 | Simulink:masks:boolean
      mask Callback ZeroCross: sl('zeroCrossEnable', gcbh);
      mask Display: disp(str)
  Constant : Constant  Value=4
  Constant3 : Constant
  Constant4 : Constant  Value=0
  Switch : Switch  Threshold=0.5
  Switch1 : Switch  Threshold=0.5
  Out_EMD1_CMD_Command : Outport
  wires:
  Compare To Constant/1(y) -> Switch1/2
  Switch/1 -> Out_EMD1_CMD_Command/1
  Constant4/1 -> Switch1/3
  Constant3/1 -> Switch1/1
  Constant/1 -> Switch/1
  Switch1/1 -> Switch/3
  Compare To Constant1/1(y) -> Switch/2
  EMD1_CMD_ClearErrors/1 -> Compare To Constant1/1(u)
  EMD1_CMD_MotorControlMode/1 -> Compare To Constant/1(u)

== system Energy_converter_Electrical_to_Mechanical/AWR_DriveEmot_edb_Data/Emot1_4 ==
  nGbxEMIn : Inport
  voltBatHV1 : Inport  Port=2
  trqEmotDesPhy1 : Inport  Port=3
  emot_CMD1 : Inport  Port=4
  voltBatHV4 : Inport  Port=5
  trqEmotDesPhy4 : Inport  Port=6
  emot_CMD4 : Inport  Port=7
  Bus Creator1 : BusCreator  Inputs=5
  Bus Creator2 : BusCreator  Inputs=5
  Bus Creator3 : BusCreator  Inputs=2
  e-Motor_edb_data : Energy_converter_Electrical_to_Mechanical/e-Motor_edb_data  SystemSampleTime=-1
  e-Motor_edb_data1 : Energy_converter_Electrical_to_Mechanical/e-Motor_edb_data  SystemSampleTime=-1
  emot1_4B : Outport
  wires:
  emot_CMD4/1 -> e-Motor_edb_data1/4
  emot_CMD1/1 -> e-Motor_edb_data/4
  e-Motor_edb_data1/5 -> Bus Creator2/5
  e-Motor_edb_data1/4 -> Bus Creator2/4
  e-Motor_edb_data1/3 -> Bus Creator2/3
  e-Motor_edb_data1/2 -> Bus Creator2/2
  e-Motor_edb_data1/1 -> Bus Creator2/1
  e-Motor_edb_data/5 -> Bus Creator1/5
  e-Motor_edb_data/2 -> Bus Creator1/2
  e-Motor_edb_data/1 -> Bus Creator1/1
  e-Motor_edb_data/4 -> Bus Creator1/4
  e-Motor_edb_data/3 -> Bus Creator1/3
  nGbxEMIn/1 -> e-Motor_edb_data/1, [nGbxEMIn]
  trqEmotDesPhy1/1 -> e-Motor_edb_data/3
  voltBatHV1/1 -> e-Motor_edb_data/2
  [nGbxEMIn] -> e-Motor_edb_data1/1
  voltBatHV4/1 -> e-Motor_edb_data1/2
  Bus Creator1/1 -> Bus Creator3/1  "emot1B"
  Bus Creator2/1 -> Bus Creator3/2  "emot4B"
  trqEmotDesPhy4/1 -> e-Motor_edb_data1/3
  Bus Creator3/1 -> emot1_4B/1  "emot1_4B"

== system Energy_converter_Electrical_to_Mechanical/AWR_DriveEmot_edb_Data/Emot2_3 ==
  nGbxEMIn : Inport
  voltBatHV2 : Inport  Port=2
  trqEmotDesPhy2 : Inport  Port=3
  emot_CMD2 : Inport  Port=4
  voltBatHV3 : Inport  Port=5
  trqEmotDesPhy3 : Inport  Port=6
  emot_CMD3 : Inport  Port=7
  Enable : EnablePort  StatesWhenEnabling=reset
  Bus Creator1 : BusCreator  Inputs=5
  Bus Creator2 : BusCreator  Inputs=5
  Bus Creator3 : BusCreator  Inputs=2
  e-Motor_edb_data : Energy_converter_Electrical_to_Mechanical/e-Motor_edb_data  SystemSampleTime=-1
  e-Motor_edb_data1 : Energy_converter_Electrical_to_Mechanical/e-Motor_edb_data  SystemSampleTime=-1
  emot2_3B : Outport
  wires:
  Bus Creator3/1 -> emot2_3B/1  "emot2_3B"
  trqEmotDesPhy3/1 -> e-Motor_edb_data1/3
  Bus Creator2/1 -> Bus Creator3/2  "emot3B"
  Bus Creator1/1 -> Bus Creator3/1  "emot2B"
  voltBatHV3/1 -> e-Motor_edb_data1/2
  [nGbxEMIn] -> e-Motor_edb_data1/1
  voltBatHV2/1 -> e-Motor_edb_data/2
  trqEmotDesPhy2/1 -> e-Motor_edb_data/3
  nGbxEMIn/1 -> e-Motor_edb_data/1, [nGbxEMIn]
  e-Motor_edb_data/3 -> Bus Creator1/3
  e-Motor_edb_data/4 -> Bus Creator1/4
  e-Motor_edb_data/1 -> Bus Creator1/1
  e-Motor_edb_data/2 -> Bus Creator1/2
  e-Motor_edb_data/5 -> Bus Creator1/5
  e-Motor_edb_data1/1 -> Bus Creator2/1
  e-Motor_edb_data1/2 -> Bus Creator2/2
  e-Motor_edb_data1/3 -> Bus Creator2/3
  e-Motor_edb_data1/4 -> Bus Creator2/4
  e-Motor_edb_data1/5 -> Bus Creator2/5
  emot_CMD2/1 -> e-Motor_edb_data/4
  emot_CMD3/1 -> e-Motor_edb_data1/4

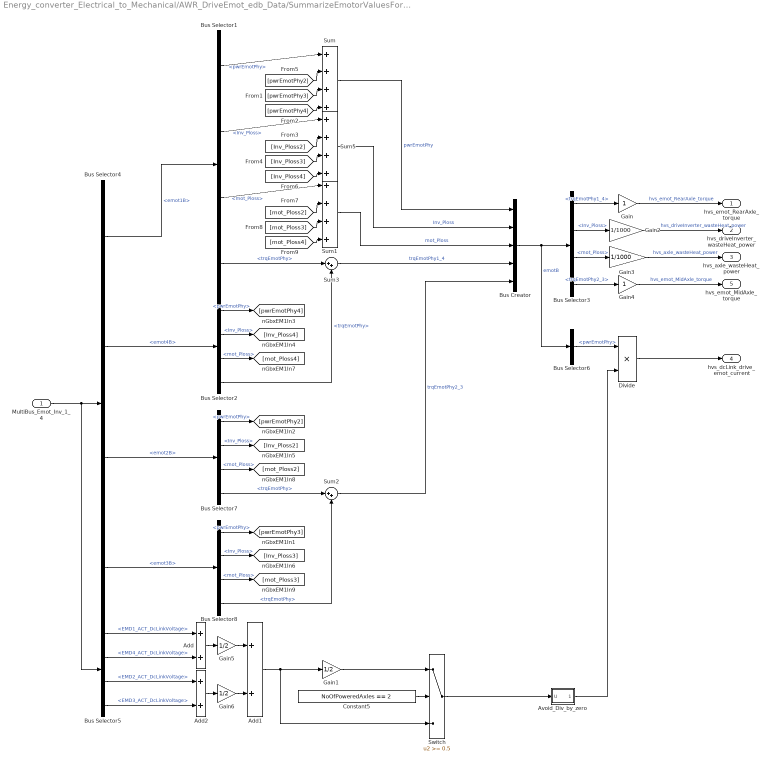
== system Energy_converter_Electrical_to_Mechanical/AWR_DriveEmot_edb_Data/SummarizeEmotorValuesForVehicle ==
  MultiBus_Emot_Inv_1_4 : Inport
  Add : Sum
  Add1 : Sum
  Add2 : Sum
  Avoid_Div_by_zero : Subsystem
  Bus Creator : BusCreator  Inputs=5
  Bus Selector{1..2,7..8} (4 alike) : BusSelector  OutputSignals=pwrEmotPhy,Inv_Ploss,mot_Ploss,trqEmotPhy
  Bus Selector3 : BusSelector  OutputSignals=trqEmotPhy1_4,Inv_Ploss,mot_Ploss,trqEmotPhy2_3
  Bus Selector4 : BusSelector  OutputSignals=emot1_4B.emot1B,emot1_4B.emot4B,emot2_3B.emot2B,emot2_3B.emot3B
  Bus Selector5 : BusSelector  OutputSignals=awr1_4B.awr1B.EMD1_ACT_DcLinkVoltage,awr1_4B.awr4B.EMD4_ACT_DcLinkVoltage,awr2_3B.awr2B.EMD2_ACT_DcLinkVoltage,awr2_3B.awr3B.EMD3_ACT_DcLinkVoltage
  Bus Selector6 : BusSelector  OutputSignals=pwrEmotPhy
  Constant5 : Constant  Value=NoOfPoweredAxles == 2
  Divide : Product  Inputs=**
  Gain : Gain
  Gain1 : Gain  Gain=1/2
  Gain2 : Gain  Gain=1/1000
  Gain3 : Gain  Gain=1/1000
  Gain4 : Gain
  Gain5 : Gain  Gain=1/2
  Gain6 : Gain  Gain=1/2
  Sum : Sum  Inputs=|++++
  Sum1 : Sum  Inputs=|++++
  Sum2 : Sum  Inputs=|++
  Sum3 : Sum  Inputs=|++
  Sum5 : Sum  Inputs=|++++
  Switch : Switch  Threshold=0.5
  hvs_emot_RearAxle_torque : Outport
  hvs_driveInverter_wasteHeat_power : Outport  Port=2
  hvs_axle_wasteHeat_power : Outport  Port=3
  hvs_dcLink_drive_emot_current : Outport  Port=4
  hvs_emot_MidAxle_torque : Outport  Port=5
  wires:
  Sum3/1 -> Bus Creator/4  "trqEmotPhy1_4"
  Sum1/1 -> Bus Creator/3  "mot_Ploss"
  Sum5/1 -> Bus Creator/2  "Inv_Ploss"
  Sum/1 -> Bus Creator/1  "pwrEmotPhy"
  Bus Selector2/4 -> Sum3/2  "<trqEmotPhy>"
  Bus Selector1/4 -> Sum3/1  "<trqEmotPhy>"
  Bus Selector2/3 -> [mot_Ploss4]  "<mot_Ploss>"
  Bus Selector1/3 -> Sum1/1  "<mot_Ploss>"
  Bus Selector2/2 -> [Inv_Ploss4]  "<Inv_Ploss>"
  Bus Selector1/2 -> Sum5/1  "<Inv_Ploss>"
  Bus Selector1/1 -> Sum/1  "<pwrEmotPhy>"
  Bus Selector4/2 -> Bus Selector2/1  "<emot4B>"
  Bus Selector4/1 -> Bus Selector1/1  "<emot1B>"
  MultiBus_Emot_Inv_1_4/1 -> Bus Selector5/1, Bus Selector4/1
  Bus Creator/1 -> Bus Selector6/1, Bus Selector3/1  "emotB"
  Bus Selector3/1 -> Gain/1  "<trqEmotPhy1_4>"
  Gain/1 -> hvs_emot_RearAxle_torque/1  "hvs_emot_RearAxle_torque"
  Bus Selector5/1 -> Add/1  "<EMD1_ACT_DcLinkVoltage>"
  Bus Selector5/2 -> Add/2  "<EMD4_ACT_DcLinkVoltage>"
  Add/1 -> Gain5/1
  Switch/1 -> Avoid_Div_by_zero/1(U)
  Bus Selector6/1 -> Divide/1  "<pwrEmotPhy>"
  Avoid_Div_by_zero/1(1/U) -> Divide/2
  Divide/1 -> hvs_dcLink_drive_emot_current/1
  Bus Selector3/2 -> Gain2/1  "<Inv_Ploss>"
  Gain2/1 -> hvs_driveInverter_wasteHeat_power/1  "hvs_driveInverter_wasteHeat_power"
  Bus Selector3/3 -> Gain3/1  "<mot_Ploss>"
  Gain3/1 -> hvs_axle_wasteHeat_power/1  "hvs_axle_wasteHeat_power"
  Bus Selector4/4 -> Bus Selector8/1  "<emot3B>"
  Bus Selector4/3 -> Bus Selector7/1  "<emot2B>"
  Bus Selector7/1 -> [pwrEmotPhy2]  "<pwrEmotPhy>"
  Bus Selector8/1 -> [pwrEmotPhy3]  "<pwrEmotPhy>"
  Bus Selector2/1 -> [pwrEmotPhy4]  "<pwrEmotPhy>"
  [pwrEmotPhy2] -> Sum/2
  [pwrEmotPhy3] -> Sum/3
  [pwrEmotPhy4] -> Sum/4
  [Inv_Ploss2] -> Sum5/2
  [Inv_Ploss3] -> Sum5/3
  [Inv_Ploss4] -> Sum5/4
  Bus Selector7/2 -> [Inv_Ploss2]  "<Inv_Ploss>"
  Bus Selector8/2 -> [Inv_Ploss3]  "<Inv_Ploss>"
  Bus Selector7/3 -> [mot_Ploss2]  "<mot_Ploss>"
  Bus Selector8/3 -> [mot_Ploss3]  "<mot_Ploss>"
  [mot_Ploss2] -> Sum1/2
  [mot_Ploss3] -> Sum1/3
  [mot_Ploss4] -> Sum1/4
  Bus Selector7/4 -> Sum2/1  "<trqEmotPhy>"
  Bus Selector8/4 -> Sum2/2  "<trqEmotPhy>"
  Sum2/1 -> Bus Creator/5  "trqEmotPhy2_3"
  Bus Selector5/3 -> Add2/1  "<EMD2_ACT_DcLinkVoltage>"
  Bus Selector5/4 -> Add2/2  "<EMD3_ACT_DcLinkVoltage>"
  Gain4/1 -> hvs_emot_MidAxle_torque/1  "hvs_emot_MidAxle_torque"
  Bus Selector3/4 -> Gain4/1  "<trqEmotPhy2_3>"
  Add2/1 -> Gain6/1
  Gain5/1 -> Add1/1
  Gain6/1 -> Add1/2
  Constant5/1 -> Switch/2
  Add1/1 -> Switch/3, Gain1/1
  Gain1/1 -> Switch/1

== system Energy_converter_Electrical_to_Mechanical/AWR_DriveEmot_edb_Data/percent_to_Nm ==
  Percentage_Torque : Inport
  Reference_Torque : Inport  Port=2
  Constant : Constant  Value=100
  Divide : Product  Inputs=*/
  Product : Product  RndMeth=Zero
  Torque_Nm : Outport
  wires:
  Constant/1 -> Divide/2
  Product/1 -> Divide/1
  Reference_Torque/1 -> Product/2  "Reference_Torque"
  Divide/1 -> Torque_Nm/1  "Torque_Nm"
  Percentage_Torque/1 -> Product/1  "Percentage_Torque"

== system Energy_converter_Electrical_to_Mechanical/AWR_DriveEmot_edb_Data/percent_to_Nm1 ==
  Percentage_Torque : Inport
  Reference_Torque : Inport  Port=2
  Constant : Constant  Value=100
  Divide : Product  Inputs=*/
  Product : Product  RndMeth=Zero
  Torque_Nm : Outport
  wires:
  Constant/1 -> Divide/2
  Product/1 -> Divide/1
  Reference_Torque/1 -> Product/2  "Reference_Torque"
  Divide/1 -> Torque_Nm/1  "Torque_Nm"
  Percentage_Torque/1 -> Product/1  "Percentage_Torque"

== system Energy_converter_Electrical_to_Mechanical/AWR_DriveEmot_edb_Data/percent_to_Nm2 ==
  Percentage_Torque : Inport
  Reference_Torque : Inport  Port=2
  Constant : Constant  Value=100
  Divide : Product  Inputs=*/
  Product : Product  RndMeth=Zero
  Torque_Nm : Outport
  wires:
  Constant/1 -> Divide/2
  Product/1 -> Divide/1
  Reference_Torque/1 -> Product/2  "Reference_Torque"
  Divide/1 -> Torque_Nm/1  "Torque_Nm"
  Percentage_Torque/1 -> Product/1  "Percentage_Torque"

== system Energy_converter_Electrical_to_Mechanical/AWR_DriveEmot_edb_Data/percent_to_Nm3 ==
  Percentage_Torque : Inport
  Reference_Torque : Inport  Port=2
  Constant : Constant  Value=100
  Divide : Product  Inputs=*/
  Product : Product  RndMeth=Zero
  Torque_Nm : Outport
  wires:
  Constant/1 -> Divide/2
  Product/1 -> Divide/1
  Reference_Torque/1 -> Product/2  "Reference_Torque"
  Divide/1 -> Torque_Nm/1  "Torque_Nm"
  Percentage_Torque/1 -> Product/1  "Percentage_Torque"

== system Energy_converter_Electrical_to_Mechanical/Emot AC Compressor Front/Avoid_Div_by_zero ==
  U : Inport
  Constant : Constant  Value=10^-6
  Divide : Product  Inputs=/*
  Math Function : Math  Operator=square  SaturateOnIntegerOverflow=on
  Sum : Sum  Inputs=++|
  1/U : Outport
  wires:
  Divide/1 -> 1/U/1
  Math Function/1 -> Divide/1
  Sum/1 -> Divide/2, Math Function/1
  Constant/1 -> Sum/1
  U/1 -> Sum/2

== system Energy_converter_Electrical_to_Mechanical/Emot AC Compressor Rear/Avoid_Div_by_zero ==
  U : Inport
  Constant : Constant  Value=10^-6
  Divide : Product  Inputs=/*
  Math Function : Math  Operator=square  SaturateOnIntegerOverflow=on
  Sum : Sum  Inputs=++|
  1/U : Outport
  wires:
  Divide/1 -> 1/U/1
  Math Function/1 -> Divide/1
  Sum/1 -> Divide/2, Math Function/1
  Constant/1 -> Sum/1
  U/1 -> Sum/2

== system Energy_converter_Electrical_to_Mechanical/Emot Air Compressor/Avoid_Div_by_zero ==
  U : Inport
  Constant : Constant  Value=10^-6
  Divide : Product  Inputs=/*
  Math Function : Math  Operator=square  SaturateOnIntegerOverflow=on
  Sum : Sum  Inputs=++|
  1/U : Outport
  wires:
  Divide/1 -> 1/U/1
  Math Function/1 -> Divide/1
  Sum/1 -> Divide/2, Math Function/1
  Constant/1 -> Sum/1
  U/1 -> Sum/2

== system Energy_converter_Electrical_to_Mechanical/GTR_Electric_machine/Thermal ==
  Total power loss : Inport
  Massflow cooling fluid : Inport  Port=2
  Bus Creator2 : BusCreator  Inputs=2
  Cooling2 : Subsystem
  c2 : Constant  Value=dat.coolingFluid.flowTemp.value
  Machine temperature[K] : Outport
  Fluid outlet temperature[K] : Outport  Port=2
  wires:
  Bus Creator2/1 -> Cooling2/2(cooling inlet)
  c2/1 -> Bus Creator2/2  "temperature [K]"
  Massflow cooling fluid/1 -> Bus Creator2/1  "mass flow [kg/s]"
  Cooling2/1(internal temperature) -> Machine temperature[K]/1  "ElecMac_tAct_K"
  Total power loss/1 -> Cooling2/1(power loss)
  Cooling2/2(fluid outlet temperature) -> Fluid outlet temperature[K]/1  "ElecMac_tActCoolingOut_K"

== system Energy_converter_Electrical_to_Mechanical/GTR_Electric_machine/local controller ==
  ElecMac_nReq_radps : Inport
  ElecMac_flgReqSwitch_B : Inport  Port=2
  ElecMac_tqReq_Nm : Inport  Port=3
  ElecMac_flowActCooling_kgps : Inport  Port=4
  sensor in : Inport  Port=5
  Bus Selector3 : BusSelector  OutputSignals=ElecMac_nAct_radps
  Bus Creator : BusCreator  Inputs=2
  Compare To Zero : simulink/Logic and Bit Operations/Compare To Zero  relop=>  OutDataTypeStr=uint8  ZeroCross=off
  Max torque : Lookup  InputValues=dat.maxtorque.speed.vec  Table=dat.maxtorque.torque.vec  LookUpMeth=Interpolation-Use End Values
  Min torque : Lookup  InputValues=dat.mintorque.speed.vec  Table=dat.mintorque.torque.vec  LookUpMeth=Interpolation-Use End Values
  PI controller : Subsystem
  Product : Product  RndMeth=Zero
  Saturation Dynamic : simulink/Discontinuities/Saturation Dynamic  OutMin=[]  OutMax=[]  OutDataTypeStr=Inherit: Same as second input  OutDataType=fixdt(1, 16)  OutScaling=2^-10  DoSatur=off
  Switch1 : Switch  Threshold=0.5  SaturateOnIntegerOverflow=on
  Switch2 : Switch  Threshold=0.5  SaturateOnIntegerOverflow=on
  Electric_speed_radps : Outport
  ctrl out : Outport  Port=2
  wires:
  Compare To Zero/1 -> Product/1
  Product/1 -> Switch2/1
  PI controller/1(Ctrl signal) -> Product/2
  Min torque/1 -> Saturation Dynamic/3
  Max torque/1 -> Saturation Dynamic/1
  Switch2/1 -> Saturation Dynamic/2
  Switch1/1 -> PI controller/1(RefSpeed), Switch2/3
  Saturation Dynamic/1 -> Bus Creator/1  "torque"
  Bus Creator/1 -> ctrl out/1
  Bus Selector3/1 -> Electric_speed_radps/1, Min torque/1, Max torque/1, PI controller/2(ActSpeed)  "<ElecMac_nAct_radps>"
  sensor in/1 -> Bus Selector3/1
  ElecMac_tqReq_Nm/1 -> Switch1/3
  ElecMac_flgReqSwitch_B/1 -> Switch1/2, Switch2/2, PI controller/3(Reset)
  ElecMac_nReq_radps/1 -> Switch1/1, Compare To Zero/1
  ElecMac_flowActCooling_kgps/1 -> Bus Creator/2

== system Energy_converter_Electrical_to_Mechanical/e-Motor/Fahrmotoren ==
  nEmot_k : Inport
  nEmot_f : Inport  Port=2
  trqEmot_k : Inport  Port=3
  trqEmot_f : Inport  Port=4
  U_DC_k : Inport  Port=5
  U_DC_f : Inport  Port=6
  mot_Ploss_lookup : Interpolation_n-D  NumberOfTableDimensions=3  Table=emot_mot_pwrLoss  ExtrapMethod=Clip  ValidIndexMayReachLast=on
      settings: InputPortMap=u0,u1,u2,u3,u4,u5
  mot_Ploss : Outport
  wires:
  mot_Ploss_lookup/1 -> mot_Ploss/1
  nEmot_f/1 -> mot_Ploss_lookup/2
  nEmot_k/1 -> mot_Ploss_lookup/1
  trqEmot_k/1 -> mot_Ploss_lookup/3
  trqEmot_f/1 -> mot_Ploss_lookup/4
  U_DC_k/1 -> mot_Ploss_lookup/5
  U_DC_f/1 -> mot_Ploss_lookup/6

== system Energy_converter_Electrical_to_Mechanical/e-Motor/Thermic_Model_Inverter ==
  P_WasteHeat_Powerstack : Inport
  T_Coolant : Inport  Port=2
  T_Powerstack : Inport  Port=3
  T_Plate : Inport  Port=4
  Add : Sum  Inputs=+-
  Add1 : Sum  Inputs=+-
  C_IGBT_and_Diode : Subsystem
  C_Plate : Subsystem
  Gain : Gain  Gain=1/inv_n_IGBT_per_Switch
  Gain2 : Gain  Gain=inv_n_IGBT_per_Switch
  R_PS-Plate : Subsystem
  R_Plate-Coolant : Subsystem
  P_Coolant : Outport
  T_Powerstack_new : Outport  Port=2
  T_Plate_new : Outport  Port=3
  wires:
  Add/1 -> C_IGBT_and_Diode/1(P_Heat_eff)
  P_WasteHeat_Powerstack/1 -> Gain/1
  Add1/1 -> C_Plate/1(P_Heat_eff)
  T_Powerstack/1 -> R_PS-Plate/1(T_IGBT), C_IGBT_and_Diode/2(T)
  C_IGBT_and_Diode/1(T_new) -> T_Powerstack_new/1
  T_Plate/1 -> R_Plate-Coolant/1(T_Plate), R_PS-Plate/2(T_Plate), C_Plate/2(T)
  C_Plate/1(T_new) -> T_Plate_new/1
  T_Coolant/1 -> R_Plate-Coolant/2(T_Coolant)
  Gain/1 -> Add/1
  Gain2/1 -> P_Coolant/1
  R_PS-Plate/1(dQ) -> Add/2, Add1/1
  R_Plate-Coolant/1(dQ) -> Add1/2, Gain2/1
